simulink model "question6_sim"  (R2022b)
settings: Solver=VariableStepAuto  StartTime=0.0  StopTime=10.0  RelTol=1e-3
values from neighbouring files (symbols this model uses):
  A = [0 1 0; 0 0 1; -1 -4 -2]    [question2.m]    (also in question2_practice.m = [0 1; -2 -3]; question6.m = [0 1 0 0; k/m b/m -k/m 0; 0 0 0 1; k/m 0 -(2*k)/m -b/m])
  b = 10    [question6.m]
  B = [0;0;2]    [question2.m]    (also in question2_practice.m = [0;0]; question6.m = [0;1/m;0;0])
  C1 = [1 0 0 0]    [question6.m]
  C2 = [0 0 1 0]    [question6.m]
  D1 = [0]    [question6.m]
  D2 = [0]    [question6.m]
  k = 2    [question6.m]
  m = 0.1    [question3.m]    (also in question6.m = 20)
  omega = 2*pi    (= 6.28318530718)    [question6.m]
settings Model: Creator=adnzw  LastModifiedBy=adnzw

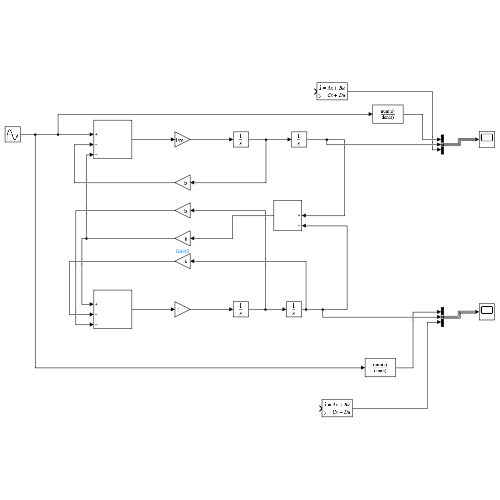
[thumbnail: Simulink's stored preview of the top-level diagram]
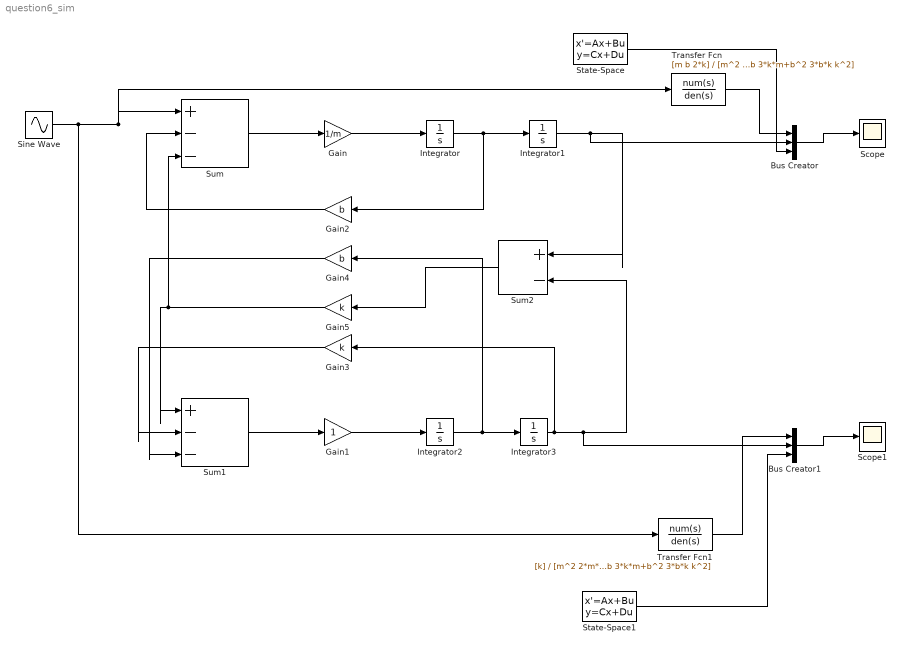
== system question6_sim ==
  Bus Creator : BusCreator  Inputs=3
  Bus Creator1 : BusCreator  Inputs=3
  Gain : Gain  Gain=1/m
  Gain1 : Gain
  Gain2 : Gain  Gain=b
  Gain3 : Gain  Gain=k
  Gain4 : Gain  Gain=b
  Gain5 : Gain  Gain=k
  Integrator{,1..3} (4 alike) : Integrator
  Scope : Scope
  Scope1 : Scope
  Sine Wave : Sin  Frequency=omega  SampleTime=0
  State-Space : StateSpace  A=A  B=B  C=C1  D=D1  InitialCondition=0
  State-Space1 : StateSpace  A=A  B=B  C=C2  D=D2  InitialCondition=0
  Sum : Sum  Inputs=|+--
  Sum1 : Sum  Inputs=|+--
  Sum2 : Sum  Inputs=|+-
  Transfer Fcn : TransferFcn  Numerator=[m b 2*k]  Denominator=[m^2 2*m*b 3*k*m+b^2 3*b*k k^2]
  Transfer Fcn1 : TransferFcn  Numerator=[k]  Denominator=[m^2 2*m*b 3*k*m+b^2 3*b*k k^2]
  wires:
  Sum/1 -> Gain/1
  Gain/1 -> Integrator/1
  Integrator/1 -> Gain2/1, Integrator1/1
  Sum1/1 -> Gain1/1
  Gain1/1 -> Integrator2/1
  Integrator2/1 -> Gain4/1, Integrator3/1
  Integrator1/1 -> Bus Creator/2, Sum2/1
  Integrator3/1 -> Gain3/1, Bus Creator1/2, Sum2/2
  Sum2/1 -> Gain5/1
  Gain5/1 -> Sum1/1, Sum/3
  Gain2/1 -> Sum/2
  Gain3/1 -> Sum1/2
  Gain4/1 -> Sum1/3
  Sine Wave/1 -> Transfer Fcn1/1, Transfer Fcn/1, Sum/1
  Bus Creator/1 -> Scope/1
  Transfer Fcn/1 -> Bus Creator/1
  Bus Creator1/1 -> Scope1/1
  Transfer Fcn1/1 -> Bus Creator1/1
  State-Space/1 -> Bus Creator/3
  State-Space1/1 -> Bus Creator1/3
